simulink model "five_pools_tcp_noise_TS_TE"  (R2018b)
settings: Solver=VariableStepAuto  StartTime=-TS/60/1000  StopTime=1440  FixedStep=(TS-TE)/60/1000  MaxStep=1/60  RelTol=1e-3
InitFcn:
  | five_pools_init_int;
  | if ~exist('SEED','var')
  |     SEED = 1;
  | end
values from neighbouring files (symbols this model uses):
  A = T*A/T    [five_pools_init_int.m]
  alpha = [6492 2478 6084 5658 7650]    [five_pools_init_int.m]
  B = T*B    [five_pools_init_int.m]
  C = eye(n)    [five_pools_init_int.m]
  D = zeros(n,n)    [five_pools_init_int.m]
  De =     [diag_trig.mat]    (also in five_pools_init_int.m = full(De); safe_sparse_trig_petc.mat = [0.62140227236 0 0 0 0 0 0 0 0 0 0.0029853512252 0 ... (225 )
  Dx =     [diag_trig.mat]    (also in safe_sparse_trig_petc.mat = [2.52853238071e-08 0 0 0 0 0 0 0 0 0 0 0 ... (225 elements, )
  epsilon = 0.000663364292932    [diag_trig.mat]    (also in safe_sparse_trig_petc.mat = 0.01)
  m = 5    [five_pools_init_int.m]
  n = 10    [five_pools_init_int.m]
  phi = [0.48 1.05 0.48 0.48 0.42]    [five_pools_init_int.m]
  SAMPLE_TIME = 60*h    (= 60)    [five_pools_init_int.m]
  tau = [4, 2, 4, 4, 6]    [five_pools_init_int.m]
  TE = 10    [five_pools_init_int.m]
  TS = 60    [five_pools_init_int.m]
  x0 = T*x0(:)    [five_pools_init_int.m]
  y0 = 0.05    [five_pools_init_int.m]
  zeta = 0.0151    [five_pools_init_int.m]
undefined symbols (not defined in the file or in its folder): f
libraries: instrumentlib x2, simulink x1
settings Model: Creator=ggleizer  LastModifiedBy=matteo
settings SolverCC: ZeroCrossControl=EnableAll
settings DebuggingCC: LibraryContextMissingDiagnostic=none
settings SFSimCC: SimUseLocalCustomCode=off
settings RTWCC: RTWUseLocalCustomCode=off

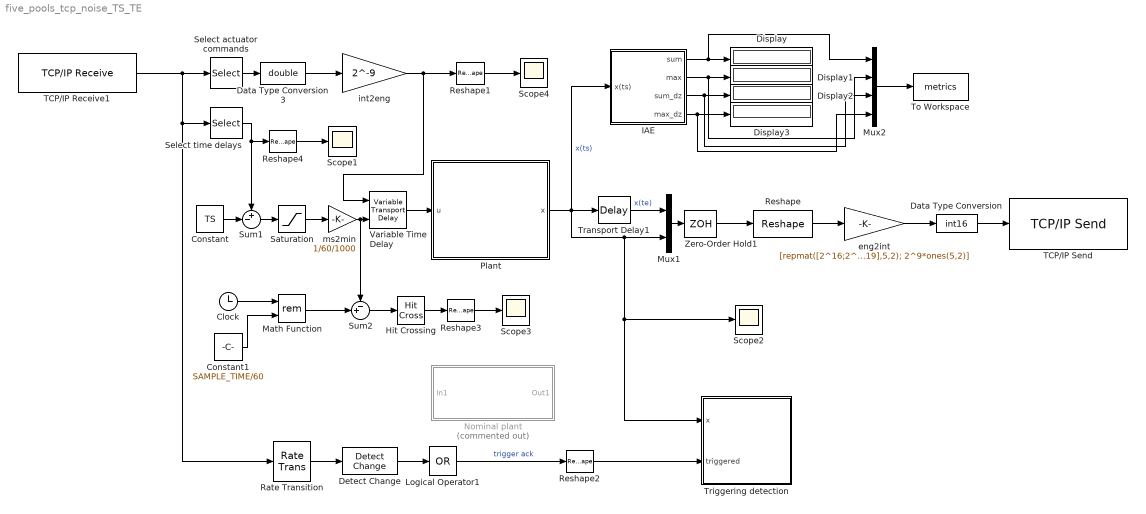
== system five_pools_tcp_noise_TS_TE ==
  Clock : Clock
  Constant : Constant  Value=TS
  Constant1 : Constant  Value=SAMPLE_TIME/60
  Data Type Conversion : DataTypeConversion  OutDataTypeStr=int16  RndMeth=Round  SaturateOnIntegerOverflow=on
  Data Type Conversion3 : DataTypeConversion  OutDataTypeStr=double  RndMeth=Round  SaturateOnIntegerOverflow=on
  Detect Change : simulink/Logic and Bit Operations/Detect Change  vinit=1  OutDataTypeStr=boolean
  Display{,1..3} (4 alike) : Display
  Hit Crossing : HitCross  HitCrossingDirection=rising
  IAE : Subsystem
  Logical Operator1 : Logic  Operator=OR  Inputs=1  AllPortsSameDT=off  OutDataTypeStr=boolean
  Math Function : Math  Operator=rem  SaturateOnIntegerOverflow=on
  Mux1 : Mux  Inputs=2
  Mux2 : Mux
  Nominal plant : Subsystem  Commented=on
  Plant : Subsystem
  Rate Transition : RateTransition  Integrity=off  Deterministic=off  OutPortSampleTime=SAMPLE_TIME/60/2
  Reshape : Reshape  OutputDimensionality=Customize  OutputDimensions=[n+5,2]
  Reshape{1..4} (4 alike) : Reshape
  Saturation : Saturate  UpperLimit=inf  LowerLimit=0
  Scope{1..4} (4 alike) : Scope
  Select actuator commands : Selector  InputPortWidth=10  IndexOptions=Index vector (dialog)  Indices=1:m  OutputSizes=1
  Select time delays : Selector  InputPortWidth=10  IndexOptions=Index vector (dialog)  Indices=m+1:2*m  OutputSizes=1
  Sum1 : Sum  Inputs=+-|
  Sum2 : Sum  Inputs=-+|
  TCP/IP Receive1 : instrumentlib/TCP//IP Receive  Priority=4  Host=localhost  Port=10020  DataSize="[10   1]"  EnableBlockingMode=on  Timeout=10  SampleTime=SAMPLE_TIME/60  DataType=int16  ByteOrder=BigEndian  ASCIIFormatting=%f,  Terminator=LF
      settings: SourceProductName=Instrument Control Toolbox
  TCP/IP Send : instrumentlib/TCP//IP Send  Priority=1  Host=localhost  Port=10021  EnableBlockingMode=off  Timeout=10  ByteOrder=BigEndian  TransferDelay=off
      settings: SourceProductName=Instrument Control Toolbox
  To Workspace : ToWorkspace  VariableName=metrics  SaveFormat=Timeseries  SampleTime=-1
      settings: MaxDataPoints=1
  Transport Delay1 : TransportDelay  DelayTime=(TS-TE)/60/1000
  Triggering detection : Subsystem
  Variable Time Delay : VariableTransportDelay  ZeroDelay=on
  Zero-Order Hold1 : ZeroOrderHold  SampleTime=SAMPLE_TIME/60
  eng2int : Gain  Gain=[repmat([2^16;2^19],5,2); 2^9*ones(5,2)]
  int2eng : Gain  Gain=2^-9
  "ms2min " : Gain  Gain=1/60/1000
  wires:
  Plant/1(x) -> IAE/1(x(ts)), Mux1/2, Scope2/1, Triggering detection/1(x), Transport Delay1/1  "x(ts)"
  TCP/IP Receive1/1 -> Rate Transition/1, Select time delays/1, Select actuator commands/1
  Transport Delay1/1 -> Mux1/1  "x(te)"
  Mux1/1 -> Zero-Order Hold1/1
  Zero-Order Hold1/1 -> Reshape/1
  Reshape/1 -> eng2int/1
  Variable Time Delay/1 -> Plant/1(u)
  Select actuator commands/1 -> Data Type Conversion3/1
  Data Type Conversion3/1 -> int2eng/1
  int2eng/1 -> Reshape1/1, Variable Time Delay/1
  Sum1/1 -> Saturation/1
  Data Type Conversion/1 -> TCP/IP Send/1
  eng2int/1 -> Data Type Conversion/1
  Constant/1 -> Sum1/2
  Select time delays/1 -> Sum1/1, Reshape4/1
  Reshape1/1 -> Scope4/1
  IAE/2(max) -> Mux2/2, Display1/1
  IAE/4(max_dz) -> Display3/1, Mux2/4
  IAE/3(sum_dz) -> Mux2/3, Display2/1
  IAE/1(sum) -> Mux2/1, Display/1
  Rate Transition/1 -> Detect Change/1
  Detect Change/1 -> Logical Operator1/1
  Logical Operator1/1 -> Reshape2/1  "trigger ack"
  Saturation/1 -> "ms2min "/1
  Mux2/1 -> To Workspace/1
  Reshape2/1 -> Triggering detection/2(triggered)
  Reshape4/1 -> Scope1/1
  Sum2/1 -> Hit Crossing/1
  Math Function/1 -> Sum2/2
  Hit Crossing/1 -> Reshape3/1
  "ms2min "/1 -> Sum2/1, Variable Time Delay/2
  Clock/1 -> Math Function/1
  Constant1/1 -> Math Function/2
  Reshape3/1 -> Scope3/1

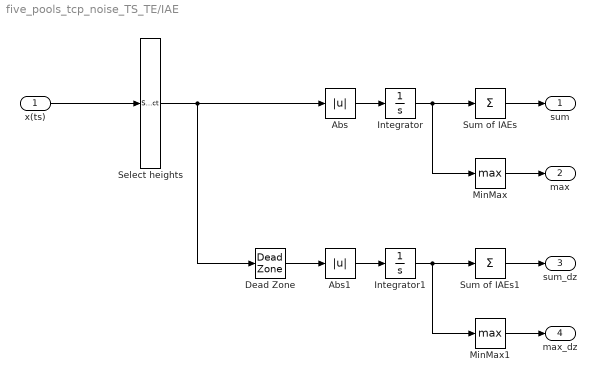
== system five_pools_tcp_noise_TS_TE/IAE ==
  x(ts) : Inport
  Abs : Abs
  Abs1 : Abs
  Dead Zone : DeadZone  LowerValue=-0.01  UpperValue=0.01  SaturateOnIntegerOverflow=on
  Integrator : Integrator
  Integrator1 : Integrator
  MinMax : MinMax  Function=max
  MinMax1 : MinMax  Function=max
  Select heights : Selector  InputPortWidth=15  IndexOptions=Index vector (dialog)  Indices=[1 3 5 7 9]  OutputSizes=1
  Sum of IAEs : Sum  Inputs=+
  Sum of IAEs1 : Sum  Inputs=+
  sum : Outport
  max : Outport  Port=2
  sum_dz : Outport  Port=3
  max_dz : Outport  Port=4
  wires:
  x(ts)/1 -> Select heights/1
  Select heights/1 -> Dead Zone/1, Abs/1
  Integrator/1 -> MinMax/1, Sum of IAEs/1
  Sum of IAEs/1 -> sum/1
  Abs/1 -> Integrator/1
  MinMax/1 -> max/1
  MinMax1/1 -> max_dz/1
  Integrator1/1 -> MinMax1/1, Sum of IAEs1/1
  Sum of IAEs1/1 -> sum_dz/1
  Dead Zone/1 -> Abs1/1
  Abs1/1 -> Integrator1/1

== system five_pools_tcp_noise_TS_TE/Nominal plant ==
  In1 : Inport
  Ground : Ground
  Mux : Mux  Inputs=2
  Mux1 : Mux  Inputs=5
  State-Space with First-order Pade approximation for time delays : StateSpace  A=A  B=B  C=C  D=D  InitialCondition=x0
  Step : Step  Time=180  After=16  SampleTime=0
  Step1 : Step  Time=450  After=18  SampleTime=0
  Step2 : Step  Time=600  After=-34  SampleTime=0
  Sum : Sum  Inputs=||+++
  Out1 : Outport
  wires:
  State-Space with First-order Pade approximation for time delays/1 -> Out1/1
  Step/1 -> Sum/1
  In1/1 -> Mux/1
  Ground/1 -> Mux1/4, Mux1/3, Mux1/2, Mux1/1
  Step1/1 -> Sum/2
  Sum/1 -> Mux1/5
  Mux1/1 -> Mux/2
  Step2/1 -> Sum/3
  Mux/1 -> State-Space with First-order Pade approximation for time delays/1

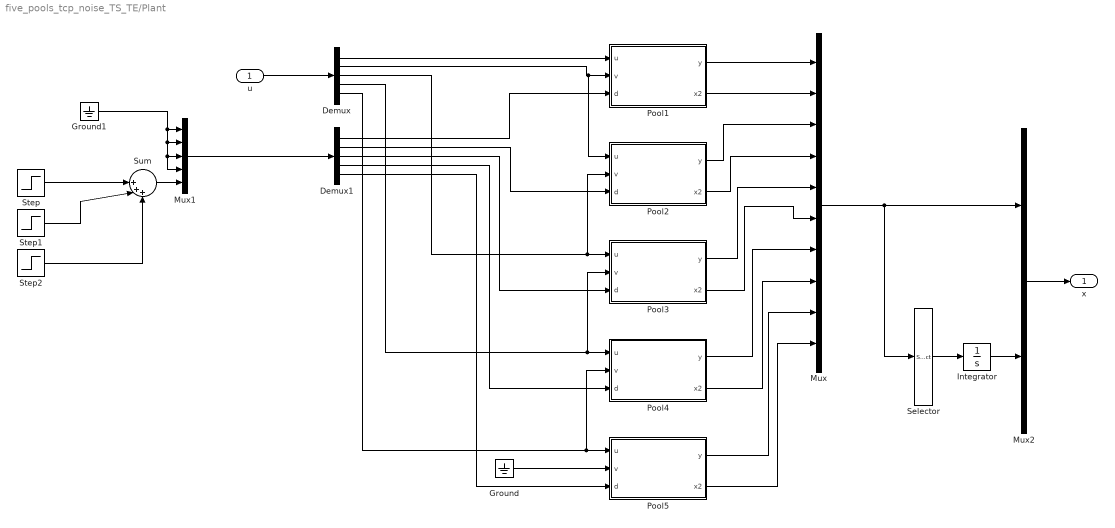
== system five_pools_tcp_noise_TS_TE/Plant ==
  u : Inport
  Demux : Demux  Outputs=5
  Demux1 : Demux  Outputs=5
  Ground : Ground
  Ground1 : Ground
  Integrator : Integrator
  Mux : Mux  Inputs=n
  Mux1 : Mux  Inputs=5
  Mux2 : Mux  Inputs=2
  Pool1 : Subsystem  mask(Pool model){y0=y0, alpha=alpha(1), tau=tau(1), phi=phi(1), zeta=zeta}
      mask prompts: y0 "Initial height (m)"; alpha "Area (m2)"; tau "Transport delay (min)"; phi "Natural frequency (rad/min)"; zeta "Damping coefficient [0,1)"
      mask help:
      | Third-order linear model of an irrigation pool.
      |   u - (linearized) gate flow in-take input
      |   v - (linearized) gate flow off-take input
      |   d - off-take disturbance
      |   y - height at the off-take side
      mask init:
      | zeta >= 0;
      | zeta < 1
      | alpha > 0;
      | tau >= 0;
      | phi >= 0;
      | omega = phi*sqrt(1 - zeta^2);
  Pool2 : Subsystem  mask(Pool model){y0=y0, alpha=alpha(2), tau=tau(2), phi=phi(2), zeta=zeta}
      mask prompts: y0 "Initial height (m)"; alpha "Area (m2)"; tau "Transport delay (min)"; phi "Natural frequency (rad/min)"; zeta "Damping coefficient [0,1)"
      mask help:
      | Third-order linear model of an irrigation pool.
      |   u - (linearized) gate flow in-take input
      |   v - (linearized) gate flow off-take input
      |   d - off-take disturbance
      |   y - height at the off-take side
      mask init:
      | zeta >= 0;
      | zeta < 1
      | alpha > 0;
      | tau >= 0;
      | phi >= 0;
      | omega = phi*sqrt(1 - zeta^2);
  Pool3 : Subsystem  mask(Pool model){y0=y0, alpha=alpha(3), tau=tau(3), phi=phi(3), zeta=zeta}
      mask prompts: y0 "Initial height (m)"; alpha "Area (m2)"; tau "Transport delay (min)"; phi "Natural frequency (rad/min)"; zeta "Damping coefficient [0,1)"
      mask help:
      | Third-order linear model of an irrigation pool.
      |   u - (linearized) gate flow in-take input
      |   v - (linearized) gate flow off-take input
      |   d - off-take disturbance
      |   y - height at the off-take side
      mask init:
      | zeta >= 0;
      | zeta < 1
      | alpha > 0;
      | tau >= 0;
      | phi >= 0;
      | omega = phi*sqrt(1 - zeta^2);
  Pool4 : Subsystem  mask(Pool model){y0=y0, alpha=alpha(4), tau=tau(4), phi=phi(4), zeta=zeta}
      mask prompts: y0 "Initial height (m)"; alpha "Area (m2)"; tau "Transport delay (min)"; phi "Natural frequency (rad/min)"; zeta "Damping coefficient [0,1)"
      mask help:
      | Third-order linear model of an irrigation pool.
      |   u - (linearized) gate flow in-take input
      |   v - (linearized) gate flow off-take input
      |   d - off-take disturbance
      |   y - height at the off-take side
      mask init:
      | zeta >= 0;
      | zeta < 1
      | alpha > 0;
      | tau >= 0;
      | phi >= 0;
      | omega = phi*sqrt(1 - zeta^2);
  Pool5 : Subsystem  mask(Pool model){y0=y0, alpha=alpha(5), tau=tau(5), phi=phi(5), zeta=zeta}
      mask prompts: y0 "Initial height (m)"; alpha "Area (m2)"; tau "Transport delay (min)"; phi "Natural frequency (rad/min)"; zeta "Damping coefficient [0,1)"
      mask help:
      | Third-order linear model of an irrigation pool.
      |   u - (linearized) gate flow in-take input
      |   v - (linearized) gate flow off-take input
      |   d - off-take disturbance
      |   y - height at the off-take side
      mask init:
      | zeta >= 0;
      | zeta < 1
      | alpha > 0;
      | tau >= 0;
      | phi >= 0;
      | omega = phi*sqrt(1 - zeta^2);
  Selector : Selector  InputPortWidth=10  IndexOptions=Index vector (dialog)  Indices=[1:2:9]  OutputSizes=1
  Step : Step  Time=180  After=16  SampleTime=0
  Step1 : Step  Time=450  After=18  SampleTime=0
  Step2 : Step  Time=600  After=-34  SampleTime=0
  Sum : Sum  Inputs=||+++
  x : Outport
  wires:
  Demux1/5 -> Pool5/3(d)
  Demux1/3 -> Pool3/3(d)
  Mux1/1 -> Demux1/1
  Demux1/2 -> Pool2/3(d)
  Ground/1 -> Pool5/2(v)
  u/1 -> Demux/1
  Demux/5 -> Pool4/2(v), Pool5/1(u)
  Demux1/4 -> Pool4/3(d)
  Demux/1 -> Pool1/1(u)
  Demux/2 -> Pool1/2(v), Pool2/1(u)
  Demux1/1 -> Pool1/3(d)
  Demux/4 -> Pool4/1(u), Pool3/2(v)
  Demux/3 -> Pool2/2(v), Pool3/1(u)
  Pool3/2(x2) -> Mux/6
  Pool4/2(x2) -> Mux/8
  Pool5/2(x2) -> Mux/10
  Pool5/1(y) -> Mux/9
  Pool4/1(y) -> Mux/7
  Pool3/1(y) -> Mux/5
  Pool1/2(x2) -> Mux/2
  Pool2/1(y) -> Mux/3
  Pool2/2(x2) -> Mux/4
  Step/1 -> Sum/1
  Sum/1 -> Mux1/5
  Ground1/1 -> Mux1/4, Mux1/3, Mux1/2, Mux1/1
  Step1/1 -> Sum/2
  Mux2/1 -> x/1
  Step2/1 -> Sum/3
  Selector/1 -> Integrator/1
  Integrator/1 -> Mux2/2
  Pool1/1(y) -> Mux/1
  Mux/1 -> Selector/1, Mux2/1

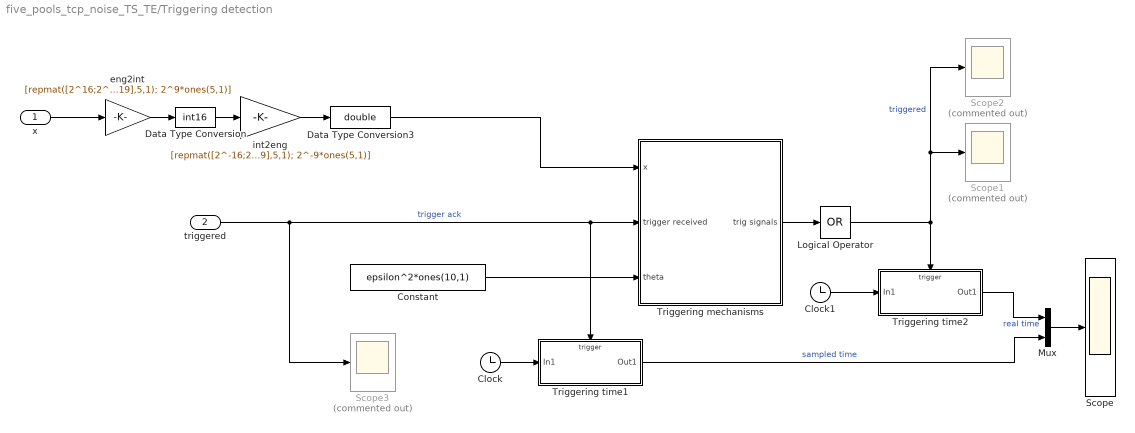
== system five_pools_tcp_noise_TS_TE/Triggering detection ==
  x : Inport
  triggered : Inport  Port=2
  Clock : Clock
  Clock1 : Clock
  Constant : Constant  Value=epsilon^2*ones(10,1)
  Data Type Conversion : DataTypeConversion  OutDataTypeStr=int16  RndMeth=Round  SaturateOnIntegerOverflow=on
  Data Type Conversion3 : DataTypeConversion  OutDataTypeStr=double
  Logical Operator : Logic  Operator=OR  Inputs=1  AllPortsSameDT=off  OutDataTypeStr=boolean
  Mux : Mux  Inputs=2
  Scope : Scope
  Scope1 : Scope  Commented=on
  Scope2 : Scope  Commented=on
  Scope3 : Scope  Commented=on
  Triggering mechanisms : Subsystem
  Triggering time1 : Subsystem  TreatAsAtomicUnit=on
  Triggering time2 : Subsystem  TreatAsAtomicUnit=on
  eng2int : Gain  Gain=[repmat([2^16;2^19],5,1); 2^9*ones(5,1)]
  int2eng : Gain  Gain=[repmat([2^-16;2^-19],5,1); 2^-9*ones(5,1)]
  wires:
  Logical Operator/1 -> Scope1/1, Scope2/1, Triggering time2/Trigger  "triggered"
  Triggering mechanisms/1("trig signals ") -> Logical Operator/1
  Constant/1 -> Triggering mechanisms/3(theta)
  triggered/1 -> Scope3/1, Triggering mechanisms/2(trigger received), Triggering time1/Trigger  "trigger ack"
  Triggering time1/1(Out1) -> Mux/2  "sampled time"
  Clock/1 -> Triggering time1/1(In1)
  eng2int/1 -> Data Type Conversion/1
  int2eng/1 -> Data Type Conversion3/1
  Data Type Conversion/1 -> int2eng/1
  x/1 -> eng2int/1
  Data Type Conversion3/1 -> Triggering mechanisms/1(x)
  Clock1/1 -> Triggering time2/1(In1)
  Mux/1 -> Scope/1
  Triggering time2/1(Out1) -> Mux/1  "real time"

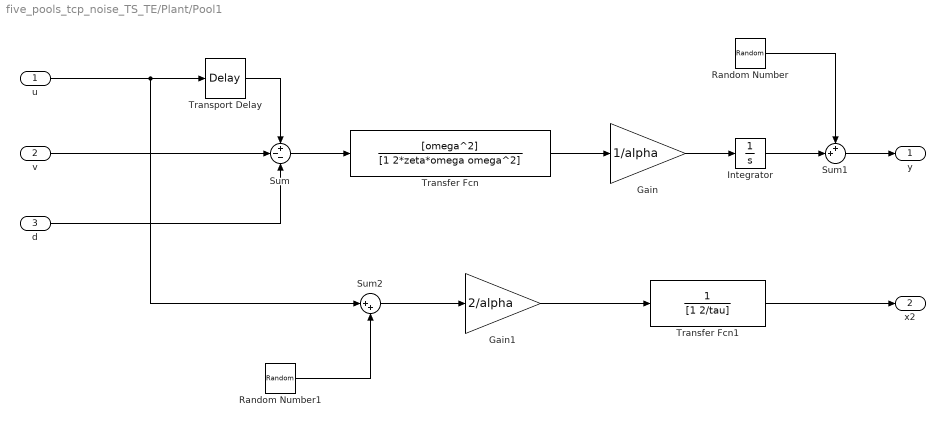
== system five_pools_tcp_noise_TS_TE/Plant/Pool1 ==
  u : Inport
  v : Inport  Port=2
  d : Inport  Port=3
  Gain : Gain  Gain=1/alpha
  Gain1 : Gain  Gain=2/alpha
  Integrator : Integrator  InitialCondition=y0
  Random Number : RandomNumber  Variance=0.001^2  Seed=SEED  SampleTime=1
  Random Number1 : RandomNumber  Variance=1^2  Seed=SEED+1  SampleTime=1
  Sum : Sum  Inputs=+--
  Sum1 : Sum  Inputs=++|
  Sum2 : Sum  Inputs=|++
  Transfer Fcn : TransferFcn  Numerator=[omega^2]  Denominator=[1 2*zeta*omega omega^2]
  Transfer Fcn1 : TransferFcn  Denominator=[1 2/tau]
  Transport Delay : TransportDelay  DelayTime=tau
  y : Outport
  x2 : Outport  Port=2
  wires:
  v/1 -> Sum/2
  d/1 -> Sum/3
  u/1 -> Sum2/1, Transport Delay/1
  Transport Delay/1 -> Sum/1
  Sum/1 -> Transfer Fcn/1
  Transfer Fcn/1 -> Gain/1
  Gain/1 -> Integrator/1
  Transfer Fcn1/1 -> x2/1
  Gain1/1 -> Transfer Fcn1/1
  Sum1/1 -> y/1
  Integrator/1 -> Sum1/2
  Sum2/1 -> Gain1/1
  Random Number/1 -> Sum1/1
  Random Number1/1 -> Sum2/2

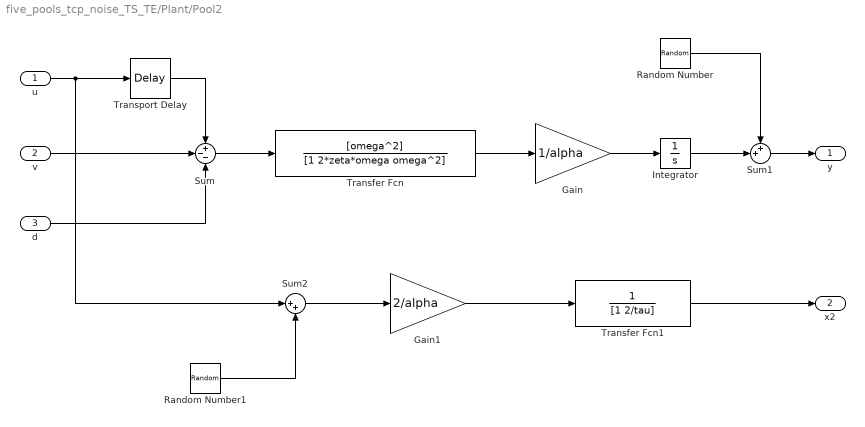
== system five_pools_tcp_noise_TS_TE/Plant/Pool2 ==
  u : Inport
  v : Inport  Port=2
  d : Inport  Port=3
  Gain : Gain  Gain=1/alpha
  Gain1 : Gain  Gain=2/alpha
  Integrator : Integrator  InitialCondition=y0
  Random Number : RandomNumber  Variance=0.001^2  Seed=SEED+2  SampleTime=1
  Random Number1 : RandomNumber  Variance=1^2  Seed=SEED+3  SampleTime=1
  Sum : Sum  Inputs=+--
  Sum1 : Sum  Inputs=++|
  Sum2 : Sum  Inputs=|++
  Transfer Fcn : TransferFcn  Numerator=[omega^2]  Denominator=[1 2*zeta*omega omega^2]
  Transfer Fcn1 : TransferFcn  Denominator=[1 2/tau]
  Transport Delay : TransportDelay  DelayTime=tau
  y : Outport
  x2 : Outport  Port=2
  wires:
  Gain/1 -> Integrator/1
  Integrator/1 -> Sum1/2
  u/1 -> Sum2/1, Transport Delay/1
  Sum1/1 -> y/1
  Sum/1 -> Transfer Fcn/1
  d/1 -> Sum/3
  Transport Delay/1 -> Sum/1
  Transfer Fcn/1 -> Gain/1
  Random Number/1 -> Sum1/1
  Transfer Fcn1/1 -> x2/1
  v/1 -> Sum/2
  Gain1/1 -> Transfer Fcn1/1
  Sum2/1 -> Gain1/1
  Random Number1/1 -> Sum2/2

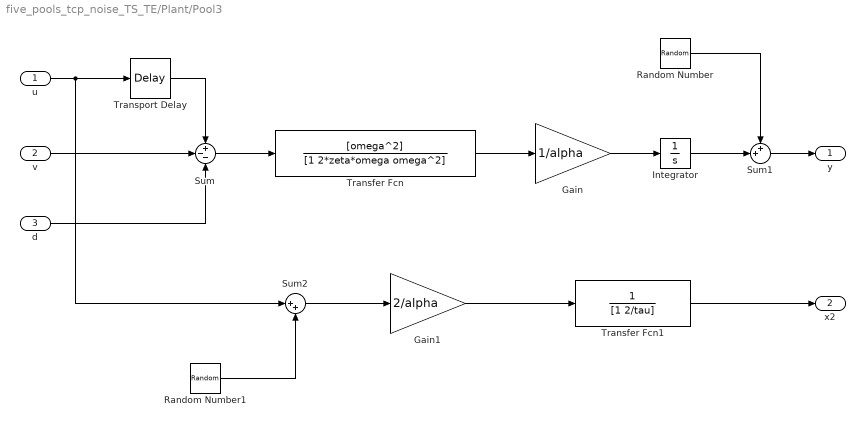
== system five_pools_tcp_noise_TS_TE/Plant/Pool3 ==
  u : Inport
  v : Inport  Port=2
  d : Inport  Port=3
  Gain : Gain  Gain=1/alpha
  Gain1 : Gain  Gain=2/alpha
  Integrator : Integrator  InitialCondition=y0
  Random Number : RandomNumber  Variance=0.001^2  Seed=SEED+4  SampleTime=1
  Random Number1 : RandomNumber  Variance=1^2  Seed=SEED+5  SampleTime=1
  Sum : Sum  Inputs=+--
  Sum1 : Sum  Inputs=++|
  Sum2 : Sum  Inputs=|++
  Transfer Fcn : TransferFcn  Numerator=[omega^2]  Denominator=[1 2*zeta*omega omega^2]
  Transfer Fcn1 : TransferFcn  Denominator=[1 2/tau]
  Transport Delay : TransportDelay  DelayTime=tau
  y : Outport
  x2 : Outport  Port=2
  wires:
  u/1 -> Sum2/1, Transport Delay/1
  Sum1/1 -> y/1
  Sum2/1 -> Gain1/1
  Gain1/1 -> Transfer Fcn1/1
  Transfer Fcn1/1 -> x2/1
  v/1 -> Sum/2
  d/1 -> Sum/3
  Random Number1/1 -> Sum2/2
  Sum/1 -> Transfer Fcn/1
  Integrator/1 -> Sum1/2
  Gain/1 -> Integrator/1
  Random Number/1 -> Sum1/1
  Transport Delay/1 -> Sum/1
  Transfer Fcn/1 -> Gain/1

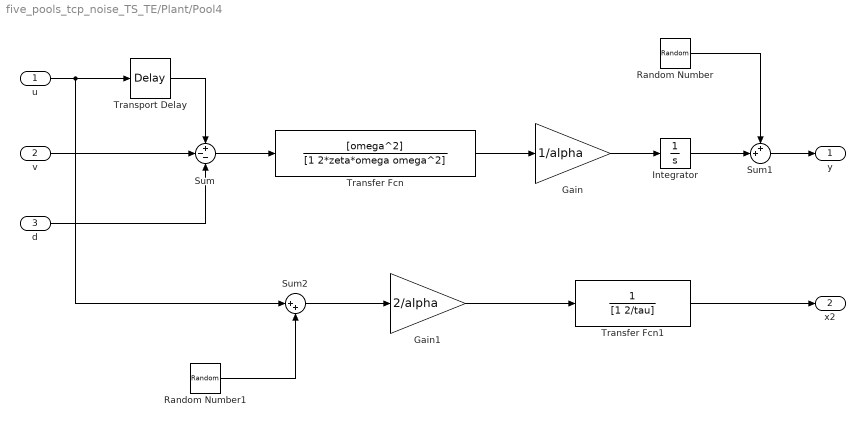
== system five_pools_tcp_noise_TS_TE/Plant/Pool4 ==
  u : Inport
  v : Inport  Port=2
  d : Inport  Port=3
  Gain : Gain  Gain=1/alpha
  Gain1 : Gain  Gain=2/alpha
  Integrator : Integrator  InitialCondition=y0
  Random Number : RandomNumber  Variance=0.001^2  Seed=SEED+6  SampleTime=1
  Random Number1 : RandomNumber  Variance=1^2  Seed=SEED+7  SampleTime=1
  Sum : Sum  Inputs=+--
  Sum1 : Sum  Inputs=++|
  Sum2 : Sum  Inputs=|++
  Transfer Fcn : TransferFcn  Numerator=[omega^2]  Denominator=[1 2*zeta*omega omega^2]
  Transfer Fcn1 : TransferFcn  Denominator=[1 2/tau]
  Transport Delay : TransportDelay  DelayTime=tau
  y : Outport
  x2 : Outport  Port=2
  wires:
  u/1 -> Sum2/1, Transport Delay/1
  Sum1/1 -> y/1
  Sum2/1 -> Gain1/1
  Gain1/1 -> Transfer Fcn1/1
  Transfer Fcn1/1 -> x2/1
  v/1 -> Sum/2
  d/1 -> Sum/3
  Random Number1/1 -> Sum2/2
  Sum/1 -> Transfer Fcn/1
  Integrator/1 -> Sum1/2
  Gain/1 -> Integrator/1
  Random Number/1 -> Sum1/1
  Transport Delay/1 -> Sum/1
  Transfer Fcn/1 -> Gain/1

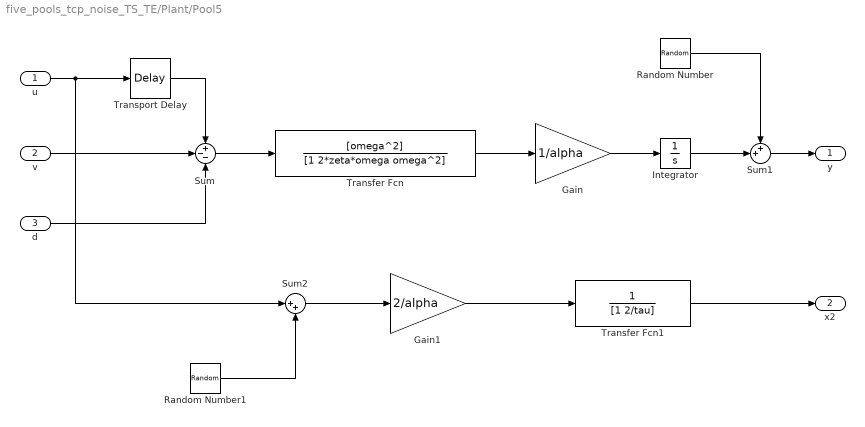
== system five_pools_tcp_noise_TS_TE/Plant/Pool5 ==
  u : Inport
  v : Inport  Port=2
  d : Inport  Port=3
  Gain : Gain  Gain=1/alpha
  Gain1 : Gain  Gain=2/alpha
  Integrator : Integrator  InitialCondition=y0
  Random Number : RandomNumber  Variance=0.001^2  Seed=SEED+8  SampleTime=SAMPLE_TIME/60
  Random Number1 : RandomNumber  Variance=1^2  Seed=SEED+9  SampleTime=SAMPLE_TIME/60
  Sum : Sum  Inputs=+--
  Sum1 : Sum  Inputs=++|
  Sum2 : Sum  Inputs=|++
  Transfer Fcn : TransferFcn  Numerator=[omega^2]  Denominator=[1 2*zeta*omega omega^2]
  Transfer Fcn1 : TransferFcn  Denominator=[1 2/tau]
  Transport Delay : TransportDelay  DelayTime=tau
  y : Outport
  x2 : Outport  Port=2
  wires:
  u/1 -> Sum2/1, Transport Delay/1
  Sum1/1 -> y/1
  Sum2/1 -> Gain1/1
  Gain1/1 -> Transfer Fcn1/1
  Transfer Fcn1/1 -> x2/1
  v/1 -> Sum/2
  d/1 -> Sum/3
  Random Number1/1 -> Sum2/2
  Sum/1 -> Transfer Fcn/1
  Integrator/1 -> Sum1/2
  Gain/1 -> Integrator/1
  Random Number/1 -> Sum1/1
  Transport Delay/1 -> Sum/1
  Transfer Fcn/1 -> Gain/1

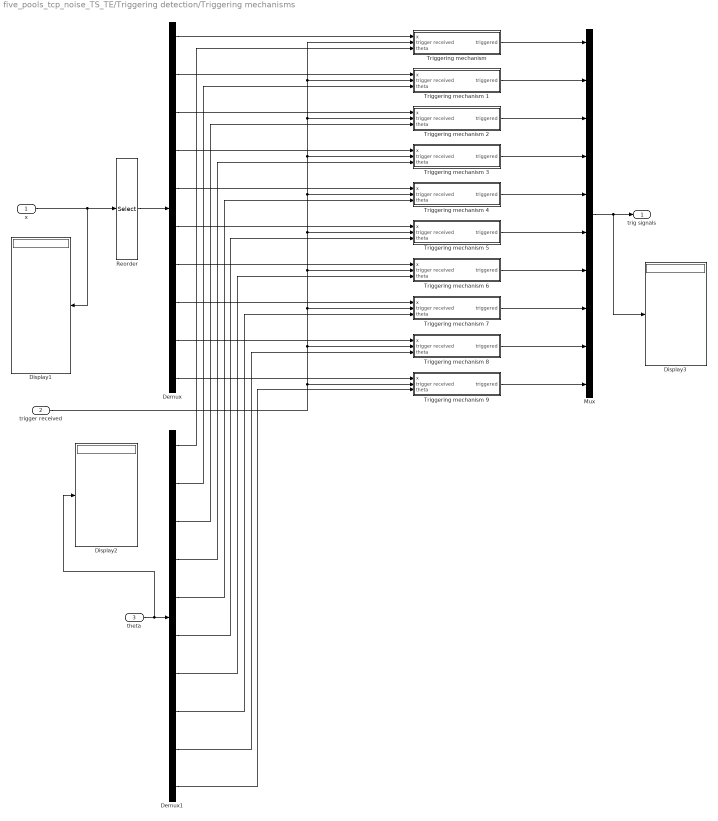
== system five_pools_tcp_noise_TS_TE/Triggering detection/Triggering mechanisms ==
  x : Inport
  trigger received : Inport  Port=2
  theta : Inport  Port=3
  Demux : Demux  Outputs=[2 2 2 2 2 1 1 1 1 1]
  Demux1 : Demux  Outputs=n
  Display1 : Display
  Display2 : Display
  Display3 : Display
  Mux : Mux  Inputs=n
  Reorder : Selector  InputPortWidth=15  IndexOptions=Index vector (dialog)  Indices=[1 11 3 12 5 13 7 14 9 15 2 4 6 8 10]  OutputSizes=1
  "Triggering mechanism " : Subsystem  mask(Triggering mechanism){De=De([1,11],[1 11]), Dx=Dx([1,11],[1 11]), x0=[0;0]}
      mask prompts: x0 "Initial state"
      mask help: Outputs held state, updating it if the following condition is satisfied: |x - \hat{x}| - sigma*|x| > epsilon, where x is the actual state, \hat{x} is the held state.
  Triggering mechanism 1 : Subsystem  mask(Triggering mechanism){De=De([3,12],[3,12]), Dx=Dx([3,12],[3,12]), x0=[0;0]}
      mask prompts: x0 "Initial state"
      mask help: Outputs held state, updating it if the following condition is satisfied: |x - \hat{x}| - sigma*|x| > epsilon, where x is the actual state, \hat{x} is the held state.
  Triggering mechanism 2 : Subsystem  mask(Triggering mechanism){De=De([5,13],[5,13]), Dx=Dx([5,13],[5,13]), x0=[0;0]}
      mask prompts: x0 "Initial state"
      mask help: Outputs held state, updating it if the following condition is satisfied: |x - \hat{x}| - sigma*|x| > epsilon, where x is the actual state, \hat{x} is the held state.
  Triggering mechanism 3 : Subsystem  mask(Triggering mechanism){De=De([7,14],[7 14]), Dx=Dx([7,14],[7 14]), x0=[0;0]}
      mask prompts: x0 "Initial state"
      mask help: Outputs held state, updating it if the following condition is satisfied: |x - \hat{x}| - sigma*|x| > epsilon, where x is the actual state, \hat{x} is the held state.
  Triggering mechanism 4 : Subsystem  mask(Triggering mechanism){De=De([9,15],[9 15]), Dx=Dx([9,15],[9 15]), x0=[0;0]}
      mask prompts: x0 "Initial state"
      mask help: Outputs held state, updating it if the following condition is satisfied: |x - \hat{x}| - sigma*|x| > epsilon, where x is the actual state, \hat{x} is the held state.
  Triggering mechanism 5 : Subsystem  mask(Triggering mechanism){De=De(2,2), Dx=Dx(2,2), x0=0}
      mask prompts: x0 "Initial state"
      mask help: Outputs held state, updating it if the following condition is satisfied: |x - \hat{x}| - sigma*|x| > epsilon, where x is the actual state, \hat{x} is the held state.
  Triggering mechanism 6 : Subsystem  mask(Triggering mechanism){De=De(4,4), Dx=Dx(4,4), x0=0}
      mask prompts: x0 "Initial state"
      mask help: Outputs held state, updating it if the following condition is satisfied: |x - \hat{x}| - sigma*|x| > epsilon, where x is the actual state, \hat{x} is the held state.
  Triggering mechanism 7 : Subsystem  mask(Triggering mechanism){De=De(6,6), Dx=Dx(6,6), x0=0}
      mask prompts: x0 "Initial state"
      mask help: Outputs held state, updating it if the following condition is satisfied: |x - \hat{x}| - sigma*|x| > epsilon, where x is the actual state, \hat{x} is the held state.
  Triggering mechanism 8 : Subsystem  mask(Triggering mechanism){De=De(8,8), Dx=Dx(8,8), x0=0}
      mask prompts: x0 "Initial state"
      mask help: Outputs held state, updating it if the following condition is satisfied: |x - \hat{x}| - sigma*|x| > epsilon, where x is the actual state, \hat{x} is the held state.
  Triggering mechanism 9 : Subsystem  mask(Triggering mechanism){De=De(10,10), Dx=Dx(10,10), x0=0}
      mask prompts: x0 "Initial state"
      mask help: Outputs held state, updating it if the following condition is satisfied: |x - \hat{x}| - sigma*|x| > epsilon, where x is the actual state, \hat{x} is the held state.
  "trig signals " : Outport
  wires:
  Demux/2 -> Triggering mechanism 1/1(x)
  Demux/1 -> "Triggering mechanism "/1(x)
  Demux/3 -> Triggering mechanism 2/1(x)
  Triggering mechanism 1/1(triggered) -> Mux/2
  "Triggering mechanism "/1(triggered) -> Mux/1
  Triggering mechanism 2/1(triggered) -> Mux/3
  Triggering mechanism 4/1(triggered) -> Mux/5
  Demux/4 -> Triggering mechanism 3/1(x)
  Demux/6 -> Triggering mechanism 5/1(x)
  Demux/5 -> Triggering mechanism 4/1(x)
  Triggering mechanism 3/1(triggered) -> Mux/4
  Triggering mechanism 5/1(triggered) -> Mux/6
  Triggering mechanism 7/1(triggered) -> Mux/8
  Demux/7 -> Triggering mechanism 6/1(x)
  Demux/9 -> Triggering mechanism 8/1(x)
  Demux/8 -> Triggering mechanism 7/1(x)
  Triggering mechanism 6/1(triggered) -> Mux/7
  Triggering mechanism 8/1(triggered) -> Mux/9
  Demux/10 -> Triggering mechanism 9/1(x)
  Triggering mechanism 9/1(triggered) -> Mux/10
  trigger received/1 -> Triggering mechanism 9/2(trigger received), Triggering mechanism 8/2(trigger received), Triggering mechanism 7/2(trigger received), Triggering mechanism 6/2(trigger received), Triggering mechanism 5/2(trigger received), Triggering mechanism 4/2(trigger received), Triggering mechanism 3/2(trigger received), Triggering mechanism 2/2(trigger received), Triggering mechanism 1/2(trigger received), "Triggering mechanism "/2(trigger received)
  Mux/1 -> Display3/1, "trig signals "/1
  theta/1 -> Display2/1, Demux1/1
  Demux1/1 -> "Triggering mechanism "/3(theta)
  Demux1/2 -> Triggering mechanism 1/3(theta)
  Demux1/3 -> Triggering mechanism 2/3(theta)
  Demux1/4 -> Triggering mechanism 3/3(theta)
  Demux1/5 -> Triggering mechanism 4/3(theta)
  Demux1/6 -> Triggering mechanism 5/3(theta)
  Demux1/7 -> Triggering mechanism 6/3(theta)
  Demux1/8 -> Triggering mechanism 7/3(theta)
  Demux1/9 -> Triggering mechanism 8/3(theta)
  Demux1/10 -> Triggering mechanism 9/3(theta)
  x/1 -> Display1/1, Reorder/1
  Reorder/1 -> Demux/1

== system five_pools_tcp_noise_TS_TE/Triggering detection/Triggering time1 ==
  In1 : Inport
  Trigger : TriggerPort  VariantControl=Variant  InitialTriggerSignalState=zero
  Out1 : Outport
  wires:
  In1/1 -> Out1/1

== system five_pools_tcp_noise_TS_TE/Triggering detection/Triggering time2 ==
  In1 : Inport
  Trigger : TriggerPort  VariantControl=Variant
  Out1 : Outport
  wires:
  In1/1 -> Out1/1

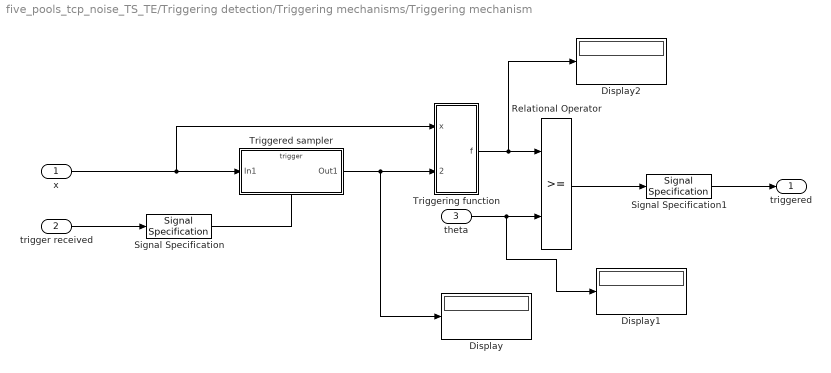
== system five_pools_tcp_noise_TS_TE/Triggering detection/Triggering mechanisms/Triggering mechanism  ==
  x : Inport
  trigger received : Inport  Port=2
  theta : Inport  Port=3
  Display : Display
  Display1 : Display
  Display2 : Display
  Relational Operator : RelationalOperator  OutDataTypeStr=boolean  RndMeth=Simplest
  Signal Specification : SignalSpecification  OutDataTypeStr=boolean
  Signal Specification1 : SignalSpecification  OutDataTypeStr=boolean
  Triggered sampler : Subsystem  TreatAsAtomicUnit=on
  Triggering function : Subsystem
  triggered : Outport
  wires:
  x/1 -> Triggered sampler/1(In1), Triggering function/1(x)
  Relational Operator/1 -> Signal Specification1/1
  Triggering function/1(f) -> Display2/1, Relational Operator/1
  trigger received/1 -> Signal Specification/1
  Signal Specification/1 -> Triggered sampler/Trigger
  Signal Specification1/1 -> triggered/1
  Triggered sampler/1(Out1) -> Display/1, Triggering function/2(xhat)
  theta/1 -> Display1/1, Relational Operator/2

== system five_pools_tcp_noise_TS_TE/Triggering detection/Triggering mechanisms/Triggering mechanism 1 ==
  x : Inport
  trigger received : Inport  Port=2
  theta : Inport  Port=3
  Relational Operator : RelationalOperator  OutDataTypeStr=boolean  RndMeth=Simplest
  Signal Specification : SignalSpecification  OutDataTypeStr=boolean
  Signal Specification1 : SignalSpecification  OutDataTypeStr=boolean
  Triggered sampler : Subsystem  TreatAsAtomicUnit=on
  Triggering function : Subsystem
  triggered : Outport
  wires:
  x/1 -> Triggered sampler/1(In1), Triggering function/1(x)
  Relational Operator/1 -> Signal Specification1/1
  Triggering function/1(f) -> Relational Operator/1
  trigger received/1 -> Signal Specification/1
  Signal Specification/1 -> Triggered sampler/Trigger
  Signal Specification1/1 -> triggered/1
  theta/1 -> Relational Operator/2
  Triggered sampler/1(Out1) -> Triggering function/2(xhat)

== system five_pools_tcp_noise_TS_TE/Triggering detection/Triggering mechanisms/Triggering mechanism 2 ==
  x : Inport
  trigger received : Inport  Port=2
  theta : Inport  Port=3
  Relational Operator : RelationalOperator  OutDataTypeStr=boolean  RndMeth=Simplest
  Signal Specification : SignalSpecification  OutDataTypeStr=boolean
  Signal Specification1 : SignalSpecification  OutDataTypeStr=boolean
  Triggered sampler : Subsystem  TreatAsAtomicUnit=on
  Triggering function : Subsystem
  triggered : Outport
  wires:
  x/1 -> Triggering function/1(x), Triggered sampler/1(In1)
  Relational Operator/1 -> Signal Specification1/1
  Triggering function/1(f) -> Relational Operator/1
  trigger received/1 -> Signal Specification/1
  Signal Specification/1 -> Triggered sampler/Trigger
  Signal Specification1/1 -> triggered/1
  theta/1 -> Relational Operator/2
  Triggered sampler/1(Out1) -> Triggering function/2(xhat)

== system five_pools_tcp_noise_TS_TE/Triggering detection/Triggering mechanisms/Triggering mechanism 3 ==
  x : Inport
  trigger received : Inport  Port=2
  theta : Inport  Port=3
  Relational Operator : RelationalOperator  OutDataTypeStr=boolean  RndMeth=Simplest
  Signal Specification : SignalSpecification  OutDataTypeStr=boolean
  Signal Specification1 : SignalSpecification  OutDataTypeStr=boolean
  Triggered sampler : Subsystem  TreatAsAtomicUnit=on
  Triggering function : Subsystem
  triggered : Outport
  wires:
  x/1 -> Triggered sampler/1(In1), Triggering function/1(x)
  Relational Operator/1 -> Signal Specification1/1
  Triggering function/1(f) -> Relational Operator/1
  trigger received/1 -> Signal Specification/1
  Signal Specification/1 -> Triggered sampler/Trigger
  Signal Specification1/1 -> triggered/1
  theta/1 -> Relational Operator/2
  Triggered sampler/1(Out1) -> Triggering function/2(xhat)

== system five_pools_tcp_noise_TS_TE/Triggering detection/Triggering mechanisms/Triggering mechanism 4 ==
  x : Inport
  trigger received : Inport  Port=2
  theta : Inport  Port=3
  Relational Operator : RelationalOperator  OutDataTypeStr=boolean  RndMeth=Simplest
  Signal Specification : SignalSpecification  OutDataTypeStr=boolean
  Signal Specification1 : SignalSpecification  OutDataTypeStr=boolean
  Triggered sampler : Subsystem  TreatAsAtomicUnit=on
  Triggering function : Subsystem
  triggered : Outport
  wires:
  x/1 -> Triggered sampler/1(In1), Triggering function/1(x)
  Relational Operator/1 -> Signal Specification1/1
  Triggering function/1(f) -> Relational Operator/1
  trigger received/1 -> Signal Specification/1
  Signal Specification/1 -> Triggered sampler/Trigger
  Signal Specification1/1 -> triggered/1
  theta/1 -> Relational Operator/2
  Triggered sampler/1(Out1) -> Triggering function/2(xhat)

== system five_pools_tcp_noise_TS_TE/Triggering detection/Triggering mechanisms/Triggering mechanism 5 ==
  x : Inport
  trigger received : Inport  Port=2
  theta : Inport  Port=3
  Relational Operator : RelationalOperator  OutDataTypeStr=boolean  RndMeth=Simplest
  Signal Specification : SignalSpecification  OutDataTypeStr=boolean
  Signal Specification1 : SignalSpecification  OutDataTypeStr=boolean
  Triggered sampler : Subsystem  TreatAsAtomicUnit=on
  Triggering function : Subsystem
  triggered : Outport
  wires:
  x/1 -> Triggered sampler/1(In1), Triggering function/1(x)
  Relational Operator/1 -> Signal Specification1/1
  Triggering function/1(f) -> Relational Operator/1
  trigger received/1 -> Signal Specification/1
  Signal Specification/1 -> Triggered sampler/Trigger
  Signal Specification1/1 -> triggered/1
  theta/1 -> Relational Operator/2
  Triggered sampler/1(Out1) -> Triggering function/2(xhat)

== system five_pools_tcp_noise_TS_TE/Triggering detection/Triggering mechanisms/Triggering mechanism 6 ==
  x : Inport
  trigger received : Inport  Port=2
  theta : Inport  Port=3
  Relational Operator : RelationalOperator  OutDataTypeStr=boolean  RndMeth=Simplest
  Signal Specification : SignalSpecification  OutDataTypeStr=boolean
  Signal Specification1 : SignalSpecification  OutDataTypeStr=boolean
  Triggered sampler : Subsystem  TreatAsAtomicUnit=on
  Triggering function : Subsystem
  triggered : Outport
  wires:
  x/1 -> Triggered sampler/1(In1), Triggering function/1(x)
  Relational Operator/1 -> Signal Specification1/1
  Triggering function/1(f) -> Relational Operator/1
  trigger received/1 -> Signal Specification/1
  Signal Specification/1 -> Triggered sampler/Trigger
  Signal Specification1/1 -> triggered/1
  theta/1 -> Relational Operator/2
  Triggered sampler/1(Out1) -> Triggering function/2(xhat)

== system five_pools_tcp_noise_TS_TE/Triggering detection/Triggering mechanisms/Triggering mechanism 7 ==
  x : Inport
  trigger received : Inport  Port=2
  theta : Inport  Port=3
  Relational Operator : RelationalOperator  OutDataTypeStr=boolean  RndMeth=Simplest
  Signal Specification : SignalSpecification  OutDataTypeStr=boolean
  Signal Specification1 : SignalSpecification  OutDataTypeStr=boolean
  Triggered sampler : Subsystem  TreatAsAtomicUnit=on
  Triggering function : Subsystem
  triggered : Outport
  wires:
  x/1 -> Triggered sampler/1(In1), Triggering function/1(x)
  Relational Operator/1 -> Signal Specification1/1
  Triggering function/1(f) -> Relational Operator/1
  trigger received/1 -> Signal Specification/1
  Signal Specification/1 -> Triggered sampler/Trigger
  Signal Specification1/1 -> triggered/1
  theta/1 -> Relational Operator/2
  Triggered sampler/1(Out1) -> Triggering function/2(xhat)

== system five_pools_tcp_noise_TS_TE/Triggering detection/Triggering mechanisms/Triggering mechanism 8 ==
  x : Inport
  trigger received : Inport  Port=2
  theta : Inport  Port=3
  Relational Operator : RelationalOperator  OutDataTypeStr=boolean  RndMeth=Simplest
  Signal Specification : SignalSpecification  OutDataTypeStr=boolean
  Signal Specification1 : SignalSpecification  OutDataTypeStr=boolean
  Triggered sampler : Subsystem  TreatAsAtomicUnit=on
  Triggering function : Subsystem
  triggered : Outport
  wires:
  x/1 -> Triggered sampler/1(In1), Triggering function/1(x)
  Relational Operator/1 -> Signal Specification1/1
  Triggering function/1(f) -> Relational Operator/1
  trigger received/1 -> Signal Specification/1
  Signal Specification/1 -> Triggered sampler/Trigger
  Signal Specification1/1 -> triggered/1
  theta/1 -> Relational Operator/2
  Triggered sampler/1(Out1) -> Triggering function/2(xhat)

== system five_pools_tcp_noise_TS_TE/Triggering detection/Triggering mechanisms/Triggering mechanism 9 ==
  x : Inport
  trigger received : Inport  Port=2
  theta : Inport  Port=3
  Relational Operator : RelationalOperator  OutDataTypeStr=boolean  RndMeth=Simplest
  Signal Specification : SignalSpecification  OutDataTypeStr=boolean
  Signal Specification1 : SignalSpecification  OutDataTypeStr=boolean
  Triggered sampler : Subsystem  TreatAsAtomicUnit=on
  Triggering function : Subsystem
  triggered : Outport
  wires:
  x/1 -> Triggered sampler/1(In1), Triggering function/1(x)
  Relational Operator/1 -> Signal Specification1/1
  Triggering function/1(f) -> Relational Operator/1
  trigger received/1 -> Signal Specification/1
  Signal Specification/1 -> Triggered sampler/Trigger
  Signal Specification1/1 -> triggered/1
  theta/1 -> Relational Operator/2
  Triggered sampler/1(Out1) -> Triggering function/2(xhat)

== system five_pools_tcp_noise_TS_TE/Triggering detection/Triggering mechanisms/Triggering mechanism /Triggered sampler ==
  In1 : Inport
  Trigger : TriggerPort  VariantControl=Variant  InitialTriggerSignalState=zero
  Out1 : Outport
  wires:
  In1/1 -> Out1/1

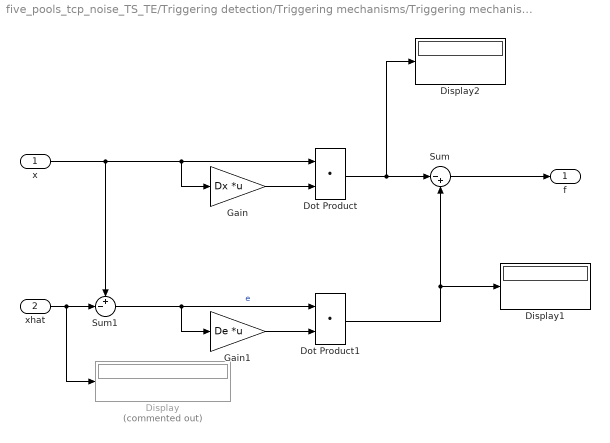
== system five_pools_tcp_noise_TS_TE/Triggering detection/Triggering mechanisms/Triggering mechanism /Triggering function ==
  x : Inport
  xhat : Inport  Port=2
  Display : Display  Commented=on
  Display1 : Display
  Display2 : Display
  Dot Product : DotProduct  InputSameDT=on  OutDataTypeStr=Inherit: Inherit via internal rule
  Dot Product1 : DotProduct  InputSameDT=on  OutDataTypeStr=Inherit: Inherit via internal rule
  Gain : Gain  Gain=Dx  Multiplication=Matrix(K*u)
  Gain1 : Gain  Gain=De  Multiplication=Matrix(K*u)
  Sum : Sum  Inputs=|-+
  Sum1 : Sum  Inputs=+-|
  f : Outport
  wires:
  xhat/1 -> Display/1, Sum1/2
  x/1 -> Gain/1, Dot Product/1, Sum1/1
  Sum1/1 -> Gain1/1, Dot Product1/1  "e"
  Sum/1 -> f/1
  Dot Product/1 -> Display2/1, Sum/1
  Gain/1 -> Dot Product/2
  Gain1/1 -> Dot Product1/2
  Dot Product1/1 -> Display1/1, Sum/2

== system five_pools_tcp_noise_TS_TE/Triggering detection/Triggering mechanisms/Triggering mechanism 1/Triggered sampler ==
  In1 : Inport
  Trigger : TriggerPort  VariantControl=Variant  InitialTriggerSignalState=zero
  Out1 : Outport
  wires:
  In1/1 -> Out1/1

== system five_pools_tcp_noise_TS_TE/Triggering detection/Triggering mechanisms/Triggering mechanism 1/Triggering function ==
  x : Inport
  xhat : Inport  Port=2
  Dot Product : DotProduct  InputSameDT=on  OutDataTypeStr=Inherit: Inherit via internal rule
  Dot Product1 : DotProduct  InputSameDT=on  OutDataTypeStr=Inherit: Inherit via internal rule
  Gain : Gain  Gain=Dx  Multiplication=Matrix(K*u)
  Gain1 : Gain  Gain=De  Multiplication=Matrix(K*u)
  Sum : Sum  Inputs=|-+
  Sum1 : Sum  Inputs=+-|
  f : Outport
  wires:
  xhat/1 -> Sum1/2
  x/1 -> Gain/1, Dot Product/1, Sum1/1
  Sum1/1 -> Gain1/1, Dot Product1/1  "e"
  Sum/1 -> f/1
  Dot Product/1 -> Sum/1
  Gain/1 -> Dot Product/2
  Gain1/1 -> Dot Product1/2
  Dot Product1/1 -> Sum/2

== system five_pools_tcp_noise_TS_TE/Triggering detection/Triggering mechanisms/Triggering mechanism 2/Triggered sampler ==
  In1 : Inport
  Trigger : TriggerPort  VariantControl=Variant  InitialTriggerSignalState=zero
  Out1 : Outport
  wires:
  In1/1 -> Out1/1

== system five_pools_tcp_noise_TS_TE/Triggering detection/Triggering mechanisms/Triggering mechanism 2/Triggering function ==
  x : Inport
  xhat : Inport  Port=2
  Display : Display  Commented=on
  Display1 : Display
  Display2 : Display
  Dot Product : DotProduct  InputSameDT=on  OutDataTypeStr=Inherit: Inherit via internal rule
  Dot Product1 : DotProduct  InputSameDT=on  OutDataTypeStr=Inherit: Inherit via internal rule
  Gain : Gain  Gain=Dx  Multiplication=Matrix(K*u)
  Gain1 : Gain  Gain=De  Multiplication=Matrix(K*u)
  Sum : Sum  Inputs=|-+
  Sum1 : Sum  Inputs=+-|
  f : Outport
  wires:
  xhat/1 -> Display/1, Sum1/2
  x/1 -> Gain/1, Dot Product/1, Sum1/1
  Sum1/1 -> Gain1/1, Dot Product1/1  "e"
  Sum/1 -> f/1
  Dot Product/1 -> Display2/1, Sum/1
  Gain/1 -> Dot Product/2
  Gain1/1 -> Dot Product1/2
  Dot Product1/1 -> Display1/1, Sum/2

== system five_pools_tcp_noise_TS_TE/Triggering detection/Triggering mechanisms/Triggering mechanism 3/Triggered sampler ==
  In1 : Inport
  Trigger : TriggerPort  VariantControl=Variant  InitialTriggerSignalState=zero
  Out1 : Outport
  wires:
  In1/1 -> Out1/1

== system five_pools_tcp_noise_TS_TE/Triggering detection/Triggering mechanisms/Triggering mechanism 3/Triggering function ==
  x : Inport
  xhat : Inport  Port=2
  Dot Product : DotProduct  InputSameDT=on  OutDataTypeStr=Inherit: Inherit via internal rule
  Dot Product1 : DotProduct  InputSameDT=on  OutDataTypeStr=Inherit: Inherit via internal rule
  Gain : Gain  Gain=Dx  Multiplication=Matrix(K*u)
  Gain1 : Gain  Gain=De  Multiplication=Matrix(K*u)
  Sum : Sum  Inputs=|-+
  Sum1 : Sum  Inputs=+-|
  f : Outport
  wires:
  xhat/1 -> Sum1/2
  x/1 -> Gain/1, Dot Product/1, Sum1/1
  Sum1/1 -> Gain1/1, Dot Product1/1  "e"
  Sum/1 -> f/1
  Dot Product/1 -> Sum/1
  Gain/1 -> Dot Product/2
  Gain1/1 -> Dot Product1/2
  Dot Product1/1 -> Sum/2

== system five_pools_tcp_noise_TS_TE/Triggering detection/Triggering mechanisms/Triggering mechanism 4/Triggered sampler ==
  In1 : Inport
  Trigger : TriggerPort  VariantControl=Variant  InitialTriggerSignalState=zero
  Out1 : Outport
  wires:
  In1/1 -> Out1/1

== system five_pools_tcp_noise_TS_TE/Triggering detection/Triggering mechanisms/Triggering mechanism 4/Triggering function ==
  x : Inport
  xhat : Inport  Port=2
  Dot Product : DotProduct  InputSameDT=on  OutDataTypeStr=Inherit: Inherit via internal rule
  Dot Product1 : DotProduct  InputSameDT=on  OutDataTypeStr=Inherit: Inherit via internal rule
  Gain : Gain  Gain=Dx  Multiplication=Matrix(K*u)
  Gain1 : Gain  Gain=De  Multiplication=Matrix(K*u)
  Sum : Sum  Inputs=|-+
  Sum1 : Sum  Inputs=+-|
  f : Outport
  wires:
  xhat/1 -> Sum1/2
  x/1 -> Gain/1, Dot Product/1, Sum1/1
  Sum1/1 -> Gain1/1, Dot Product1/1  "e"
  Sum/1 -> f/1
  Dot Product/1 -> Sum/1
  Gain/1 -> Dot Product/2
  Gain1/1 -> Dot Product1/2
  Dot Product1/1 -> Sum/2

== system five_pools_tcp_noise_TS_TE/Triggering detection/Triggering mechanisms/Triggering mechanism 5/Triggered sampler ==
  In1 : Inport
  Trigger : TriggerPort  VariantControl=Variant  InitialTriggerSignalState=zero
  Out1 : Outport
  wires:
  In1/1 -> Out1/1

== system five_pools_tcp_noise_TS_TE/Triggering detection/Triggering mechanisms/Triggering mechanism 5/Triggering function ==
  x : Inport
  xhat : Inport  Port=2
  Dot Product : DotProduct  InputSameDT=on  OutDataTypeStr=Inherit: Inherit via internal rule
  Dot Product1 : DotProduct  InputSameDT=on  OutDataTypeStr=Inherit: Inherit via internal rule
  Gain : Gain  Gain=Dx  Multiplication=Matrix(K*u)
  Gain1 : Gain  Gain=De  Multiplication=Matrix(K*u)
  Sum : Sum  Inputs=|-+
  Sum1 : Sum  Inputs=+-|
  f : Outport
  wires:
  xhat/1 -> Sum1/2
  x/1 -> Gain/1, Dot Product/1, Sum1/1
  Sum1/1 -> Gain1/1, Dot Product1/1  "e"
  Sum/1 -> f/1
  Dot Product/1 -> Sum/1
  Gain/1 -> Dot Product/2
  Gain1/1 -> Dot Product1/2
  Dot Product1/1 -> Sum/2

== system five_pools_tcp_noise_TS_TE/Triggering detection/Triggering mechanisms/Triggering mechanism 6/Triggered sampler ==
  In1 : Inport
  Trigger : TriggerPort  VariantControl=Variant  InitialTriggerSignalState=zero
  Out1 : Outport
  wires:
  In1/1 -> Out1/1

== system five_pools_tcp_noise_TS_TE/Triggering detection/Triggering mechanisms/Triggering mechanism 6/Triggering function ==
  x : Inport
  xhat : Inport  Port=2
  Dot Product : DotProduct  InputSameDT=on  OutDataTypeStr=Inherit: Inherit via internal rule
  Dot Product1 : DotProduct  InputSameDT=on  OutDataTypeStr=Inherit: Inherit via internal rule
  Gain : Gain  Gain=Dx  Multiplication=Matrix(K*u)
  Gain1 : Gain  Gain=De  Multiplication=Matrix(K*u)
  Sum : Sum  Inputs=|-+
  Sum1 : Sum  Inputs=+-|
  f : Outport
  wires:
  xhat/1 -> Sum1/2
  x/1 -> Gain/1, Dot Product/1, Sum1/1
  Sum1/1 -> Gain1/1, Dot Product1/1  "e"
  Sum/1 -> f/1
  Dot Product/1 -> Sum/1
  Gain/1 -> Dot Product/2
  Gain1/1 -> Dot Product1/2
  Dot Product1/1 -> Sum/2

== system five_pools_tcp_noise_TS_TE/Triggering detection/Triggering mechanisms/Triggering mechanism 7/Triggered sampler ==
  In1 : Inport
  Trigger : TriggerPort  VariantControl=Variant  InitialTriggerSignalState=zero
  Out1 : Outport
  wires:
  In1/1 -> Out1/1

== system five_pools_tcp_noise_TS_TE/Triggering detection/Triggering mechanisms/Triggering mechanism 7/Triggering function ==
  x : Inport
  xhat : Inport  Port=2
  Dot Product : DotProduct  InputSameDT=on  OutDataTypeStr=Inherit: Inherit via internal rule
  Dot Product1 : DotProduct  InputSameDT=on  OutDataTypeStr=Inherit: Inherit via internal rule
  Gain : Gain  Gain=Dx  Multiplication=Matrix(K*u)
  Gain1 : Gain  Gain=De  Multiplication=Matrix(K*u)
  Sum : Sum  Inputs=|-+
  Sum1 : Sum  Inputs=+-|
  f : Outport
  wires:
  xhat/1 -> Sum1/2
  x/1 -> Gain/1, Dot Product/1, Sum1/1
  Sum1/1 -> Gain1/1, Dot Product1/1  "e"
  Sum/1 -> f/1
  Dot Product/1 -> Sum/1
  Gain/1 -> Dot Product/2
  Gain1/1 -> Dot Product1/2
  Dot Product1/1 -> Sum/2

== system five_pools_tcp_noise_TS_TE/Triggering detection/Triggering mechanisms/Triggering mechanism 8/Triggered sampler ==
  In1 : Inport
  Trigger : TriggerPort  VariantControl=Variant  InitialTriggerSignalState=zero
  Out1 : Outport
  wires:
  In1/1 -> Out1/1

== system five_pools_tcp_noise_TS_TE/Triggering detection/Triggering mechanisms/Triggering mechanism 8/Triggering function ==
  x : Inport
  xhat : Inport  Port=2
  Dot Product : DotProduct  InputSameDT=on  OutDataTypeStr=Inherit: Inherit via internal rule
  Dot Product1 : DotProduct  InputSameDT=on  OutDataTypeStr=Inherit: Inherit via internal rule
  Gain : Gain  Gain=Dx  Multiplication=Matrix(K*u)
  Gain1 : Gain  Gain=De  Multiplication=Matrix(K*u)
  Sum : Sum  Inputs=|-+
  Sum1 : Sum  Inputs=+-|
  f : Outport
  wires:
  xhat/1 -> Sum1/2
  x/1 -> Gain/1, Dot Product/1, Sum1/1
  Sum1/1 -> Gain1/1, Dot Product1/1  "e"
  Sum/1 -> f/1
  Dot Product/1 -> Sum/1
  Gain/1 -> Dot Product/2
  Gain1/1 -> Dot Product1/2
  Dot Product1/1 -> Sum/2

== system five_pools_tcp_noise_TS_TE/Triggering detection/Triggering mechanisms/Triggering mechanism 9/Triggered sampler ==
  In1 : Inport
  Trigger : TriggerPort  VariantControl=Variant  InitialTriggerSignalState=zero
  Out1 : Outport
  wires:
  In1/1 -> Out1/1

== system five_pools_tcp_noise_TS_TE/Triggering detection/Triggering mechanisms/Triggering mechanism 9/Triggering function ==
  x : Inport
  xhat : Inport  Port=2
  Dot Product : DotProduct  InputSameDT=on  OutDataTypeStr=Inherit: Inherit via internal rule
  Dot Product1 : DotProduct  InputSameDT=on  OutDataTypeStr=Inherit: Inherit via internal rule
  Gain : Gain  Gain=Dx  Multiplication=Matrix(K*u)
  Gain1 : Gain  Gain=De  Multiplication=Matrix(K*u)
  Sum : Sum  Inputs=|-+
  Sum1 : Sum  Inputs=+-|
  f : Outport
  wires:
  xhat/1 -> Sum1/2
  x/1 -> Gain/1, Dot Product/1, Sum1/1
  Sum1/1 -> Gain1/1, Dot Product1/1  "e"
  Sum/1 -> f/1
  Dot Product/1 -> Sum/1
  Gain/1 -> Dot Product/2
  Gain1/1 -> Dot Product1/2
  Dot Product1/1 -> Sum/2
